simulink model "sf_gen"  (Simulink 7.3)
settings: Solver=ode45  StartTime=0.0  StopTime=10.0  RelTol=1e-3
settings Model: Creator=zhan  LastModifiedBy=zhan
settings DataIOCC: FinalStateName=XF  SaveFinalState=on  SaveCompleteFinalSimState=on  SaveFormat=StructureWithTime

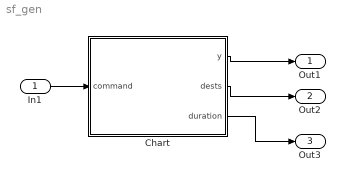
== system sf_gen ==
  In1 : Inport  OutDataType=fixdt(1, 16)  OutScaling=2^0
  Chart : Stateflow chart
  Out1 : Outport  OutDataType=fixdt(1, 16)  OutScaling=2^0
  Out2 : Outport  Port=2  OutDataType=fixdt(1, 16)  OutScaling=2^0
  Out3 : Outport  Port=3  OutDataType=fixdt(1, 16)  OutScaling=2^0
  wires:
  Chart/1(y) -> Out1/1
  In1/1 -> Chart/1(command)
  Chart/2(dests) -> Out2/1
  Chart/3(duration) -> Out3/1

== stateflow chart Chart ==
  settings: updateMethod=DISCRETE  sampleTime=0.1
  state Constant
    entry:
    dests = 2;
    duration = 4;
    during:
  state Down
    entry:
    dests=1;
    duration = 2;
    during:
    y = y-1;
    exit:
    y = y-1;
  state Up
    entry:
    dests=1;
    duration=1;
    during:
    y = y+1;
    exit:
    y = y+1;
  Constant -> Up [order 1] : after(duration*10,tick)
      | [command==1]
  Up -> Constant : after(duration*10, tick)
      | [command==1]
  Constant -> Down [order 2] : after(duration*10,tick)
      | [command==2]
  Down -> Constant : after(duration*10,tick)
      | [command==1]
  (default) -> Constant : /y = 50;
  data: y output double size=1; command input double; dests output double; duration output double
